simulink model "digitalProject"  (R2020b)
settings: Solver=FixedStepAuto  StartTime=0.0  StopTime=inf  RelTol=1e-3  EnableMultiTasking=on
libraries: arduinolib x6, arduinosensorlib x1
settings Model: SimulationMode=external  SILPILModeSetting=veronly  ExtModeTrigDuration=2  Creator=ahmed  LastModifiedBy=10
settings OptimizationCC: EnhancedBackFolding=on  PassReuseOutputArgsAs=Individual arguments  ZeroExternalMemoryAtStartup=off  ZeroInternalMemoryAtStartup=off  MaxStackSize=64  OptimizeBlockOrder=speed  DifferentSizesBufferReuse=on  OptimizationCustomize=off  EfficientTunableParamExpr=on
settings DebuggingCC: ParameterTunabilityLossMsg=error  SFMachineParentedDataDiag=error
settings HardwareCC: ProdBitPerInt=16  ProdBitPerPointer=16  ProdBitPerSizeT=16  ProdBitPerPtrDiffT=16  ProdLargestAtomicFloat=None  ProdWordSize=8  ProdHWDeviceType=Atmel->AVR
settings SFSimCC: MATLABDynamicMemAlloc=off
settings RTWCC: Description=Embedded Coder  SystemTargetFile=ert.tlc  HardwareBoard=Arduino Uno  TemplateMakefile=ert_default_tmf  Toolchain=Arduino AVR  BuildConfiguration=Faster Runs
settings CodeAppCC: ForceParamTrailComments=on  IgnoreCustomStorageClasses=off  OperatorAnnotations=on  SimulinkDataObjDesc=on  SFDataObjDesc=on  InsertBlockDesc=on
settings ERTTargetCC: SupportContinuousTime=on  SupportVariableSizeSignals=on  ExtMode=on  ExtModeStaticAllocSize=250  ExtModeMexArgs='127.0.0.1' 0 17725

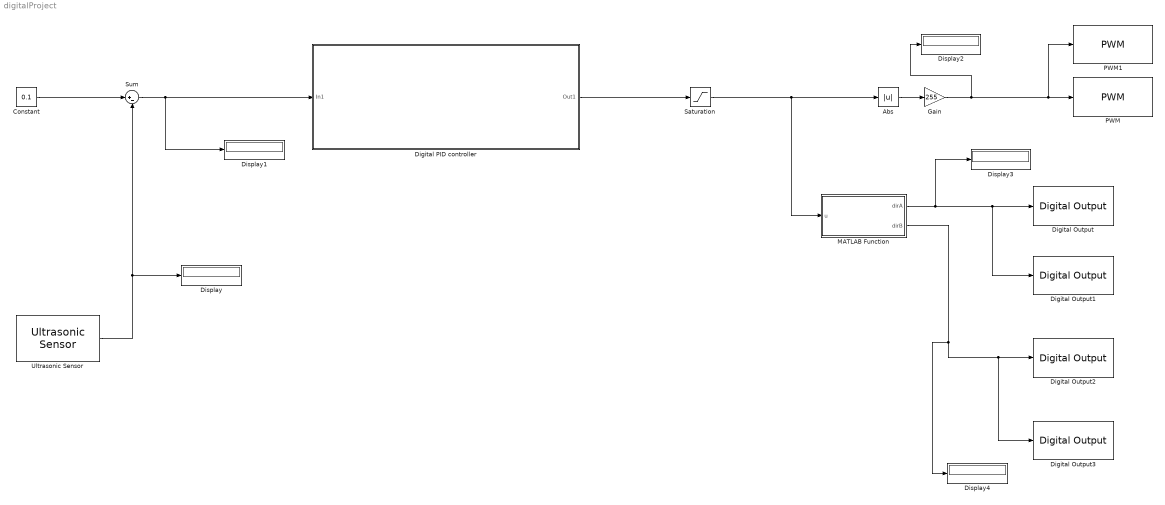
== system digitalProject ==
  Abs : Abs
  Constant : Constant  Value=0.1
  Digital Output : arduinolib/Digital Output  pinNumber=8  Direction=output  blockPlatform=arduino
  Digital Output1 : arduinolib/Digital Output  pinNumber=9  Direction=output  blockPlatform=arduino
  Digital Output2 : arduinolib/Digital Output  pinNumber=10  Direction=output  blockPlatform=arduino
  Digital Output3 : arduinolib/Digital Output  pinNumber=11  Direction=output  blockPlatform=arduino
  Digital PID controller : Subsystem
  Display{,1..4} (5 alike) : Display
  Gain : Gain  Gain=255
  MATLAB Function : MATLAB Function  TreatAsAtomicUnit=on  SystemSampleTime=0.01
  PWM : arduinolib/PWM  pinNumber=5  frequencyType=Default  desiredFrequency=490.2  achievableFrequency=490.2
  PWM1 : arduinolib/PWM  pinNumber=6  frequencyType=Default  desiredFrequency=490.2  achievableFrequency=490.2
  Saturation : Saturate  UpperLimit=1  LowerLimit=-1
  Sum : Sum  Inputs=|+-
  Ultrasonic Sensor : arduinosensorlib/Ultrasonic Sensor  NumSignalPins=2  TrigPin=2  EchoPin=3  SignalPin=3  SampleTime_=0.1  blockPlatform=ARDUINO
      settings: SourceProductBaseCode=ARDUINO
  wires:
  Constant/1 -> Sum/1
  Ultrasonic Sensor/1 -> Display/1, Sum/2
  Sum/1 -> Display1/1, Digital PID controller/1(In1)
  Abs/1 -> Gain/1
  Digital PID controller/1(Out1) -> Saturation/1
  Saturation/1 -> MATLAB Function/1(u), Abs/1
  Gain/1 -> Display2/1, PWM1/1, PWM/1
  MATLAB Function/1(dirA) -> Display3/1, Digital Output1/1, Digital Output/1
  MATLAB Function/2(dirB) -> Display4/1, Digital Output3/1, Digital Output2/1

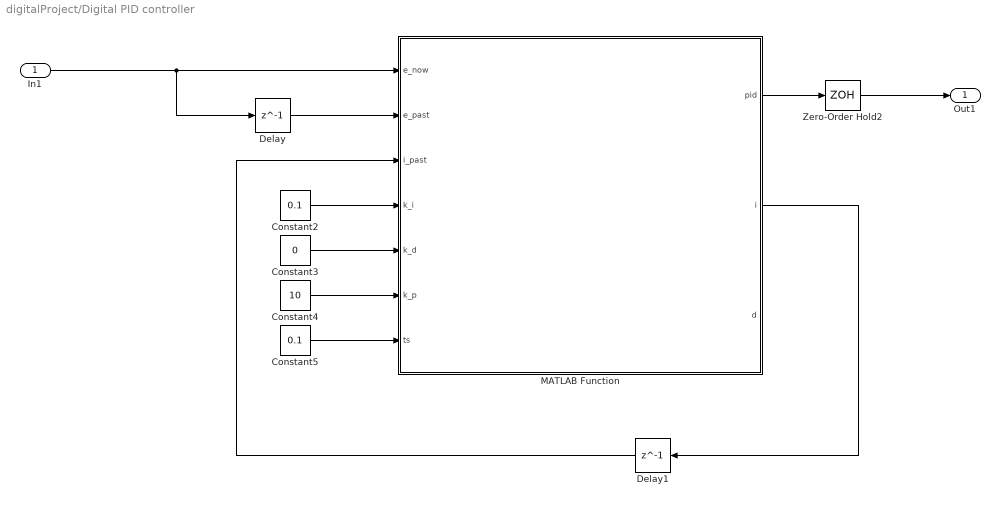
== system digitalProject/Digital PID controller ==
  In1 : Inport
  Constant2 : Constant  Value=0.1
  Constant3 : Constant  Value=0
  Constant4 : Constant  Value=10
  Constant5 : Constant  Value=0.1
  Delay : Delay  DelayLength=1  SampleTime=0.1
  Delay1 : Delay  DelayLength=1  SampleTime=0.01
  MATLAB Function : MATLAB Function  TreatAsAtomicUnit=on
  Zero-Order Hold2 : ZeroOrderHold  SampleTime=0.0001
  Out1 : Outport
  wires:
  MATLAB Function/2(i) -> Delay1/1
  Constant3/1 -> MATLAB Function/5(k_d)
  Constant4/1 -> MATLAB Function/6(k_p)
  Delay1/1 -> MATLAB Function/3(i_past)
  Constant5/1 -> MATLAB Function/7(ts)
  Constant2/1 -> MATLAB Function/4(k_i)
  In1/1 -> Delay/1, MATLAB Function/1(e_now)
  Zero-Order Hold2/1 -> Out1/1
  Delay/1 -> MATLAB Function/2(e_past)
  MATLAB Function/1(pid) -> Zero-Order Hold2/1

== matlab function digitalProject/Digital PID controller/MATLAB Function ==
  data: e_now input; e_past input; pid output; i_past input; k_i input; k_d input; k_p input; ts input; i output; d output
function [pid,i,d] = PID(e_now,e_past,i_past,k_i,k_d,k_p,ts)

d= (e_now-e_past)/ts;

i= (ts*e_now + i_past);

pid= (k_i*i) + (k_d*d) + (e_now*k_p);



end

== matlab function digitalProject/MATLAB Function ==
  data: u input; dirA output; dirB output
function [dirA,dirB] = direction(u)

if u<0
    dirA=1; dirB=0;  
elseif u>0 
    dirA=0; dirB=1;
else
    dirA=0; dirB=0;
end
